simulink model "DIMR_ordinary"  (R2024b)
settings: Solver=daessc  StartTime=0.0  StopTime=60  RelTol=1e-3
values from neighbouring files (symbols this model uses):
  d_m0 = d_mn    (= 0)    [DIMR_main.m]
  d_m_cmd = 0.12787808985686    (= 0.127878089857)    [DIMR_main.m]
  dis_cmd = 0    [DIMR_main.m]
  jrk_cmd = 0.15    [DIMR_main.m]
  phi_cmd = 0*pi/180    (= 0)    [DIMR_main.m]
  ta = (vel_cmd-jrk_cmd*tt^2)/acc_cmd    (= 3.66666666667)    [DIMR_main.m]
  taz = z_vel_cmd/z_acc_cmd    (= 1.6)    [DIMR_main.m]
  tc = (x_cmd-2*(1/2*acc_cmd*ta^2+1/2*jrk_cmd*tt^2*ta+tt*vel_cmd))/vel_cmd    (= 10.6666666667)    [DIMR_main.m]
  tcz = (z_cmd-z_acc_cmd*taz^2)/z_vel_cmd    [DIMR_main.m]
  tcz2 = (z_cmd2-z_acc_cmd*taz^2)/z_vel_cmd    (= 0.9)    [DIMR_main.m]
  theta_f0 = -theta_p0    (= -0.024)    [DIMR_main.m]
  theta_f_cmd = 0.037940459    [DIMR_main.m]
  theta_p0 = theta_pn    (= 0.024)    [DIMR_main.m]
  theta_p_cmd = -0.037940459    [DIMR_main.m]
  ts = 15    [DIMR_main.m]
  ts2 = te+5    (= 39.3333333333)    [DIMR_main.m]
  tsz = 10    [DIMR_main.m]
  tsz2 = ts2    (= 39.3333333333)    [DIMR_main.m]
  tt = acc_cmd/jrk_cmd    (= 0.333333333333)    [DIMR_main.m]
  x_cmd = 3    [DIMR_main.m]
  z_0 = R_wo+L_bmy+L_my/2    [DIMR_main.m]
  z_acc_cmd = 0.05    [DIMR_main.m]
  z_cmd = 0.9-z_0    [DIMR_main.m]
  z_cmd2 = 0.9-0.7    (= 0.2)    [DIMR_main.m]
undefined symbols (not defined in the file or in its folder): Ac, Dc, DiscIntNeverNeededParam, dspblkCoreblockFVToolHelper, g, g_ext, g_fork, g_lift, g_reac, g_spado, g_yaw, gcbh, K_fd, K_fp, K_md, K_mp, K_pd, K_pp, K_wd, K_wi, K_wp, K_yd, K_yp, Kc, L_bg, L_bmx, L_bmy, L_bmz, L_bsx, L_bsy, L_bsz, L_by, L_ex, L_ey, L_ez, L_fg, L_fh, L_fx, L_fy, L_fz, L_lx, L_ly, L_lz, L_mg, L_mx, L_my, L_mz, L_wt, M_b, M_f, M_m, M_n11, M_n21, M_n22, M_n33, M_n44, Mc, N_f, N_w, omega_c ... (+10)
libraries: simulink x56, sm_lib x54, nesl_utility x12, slctrl_autotuning x1, slpidlib x1
(part 5 of 6)

== matlab function DIMR_ordinary/IK ==
  data: dz input; mass_l input; tau input; z input; ik_theta1 output; ik_delta2 output; ik_dtheta1 output; ik_ddelta2 output; ik_lt output
function [ik_theta1,ik_delta2,ik_dtheta1,ik_ddelta2,ik_lt] = IK(dz,mass_l,tau,z)
%#codegen

%    This function was generated by the Symbolic Math Toolbox version 24.2.
%    16-Apr-2025 15:03:47

% dz = complex(dz);  % if required to enforce complex operations
% mass_l = complex(mass_l);  % if required to enforce complex operations
% tau = complex(tau);  % if required to enforce complex operations
% z = complex(z);  % if required to enforce complex operations
t0 = roots([1.0,(mass_l.*3.312391896431465e+18-z.*1.104130632143822e+21-mass_l.*z.*4.416522528575287e+19+3.992701985426881e+20)./(tau.*2.251799813685248e+18+1.700361173501486e+19),0.0,-(mass_l.*-3.312391896431465e+18+z.*1.104130632143822e+21+mass_l.*z.*4.416522528575287e+19+2.336506037211149e+20)./(tau.*2.251799813685248e+18+1.700361173501486e+19),-1.0]);
t2 = real(t0(4));
t3 = atan(t2);
t4 = mass_l.^2;
t5 = mass_l.^3;
t7 = mass_l.^5;
t9 = t2.^2;
t10 = t2.^3;
t11 = tau.^2;
t12 = tau.^3;
t14 = tau.^5;
t16 = z.^2;
t17 = z.^3;
t19 = z.^5;
t22 = mass_l+2.5e+1;
t23 = -z;
t28 = mass_l.*z.*8.0e+3;
t30 = z.*2.0e+5;
t31 = mass_l+6.81e+2./1.0e+1;
t34 = tau.*5.62949953421312e+16;
t74 = mass_l.*tau.*3.614848010623563e+119;
t84 = mass_l.*1.568588020367706e+121;
t93 = tau.*1.348008262122411e+121;
t111 = tau.*z.*1.204949336874521e+122;
t116 = mass_l.*tau.*z.*9.823967899402039e+120;
t117 = z.*5.22862673455902e+123;
t120 = mass_l.*z.*3.628335485502499e+122;
t6 = t4.^2;
t8 = t4.^3;
t13 = t11.^2;
t15 = t11.^3;
t18 = t16.^2;
t20 = t16.^3;
t21 = t3.*2.0;
ik_theta1 = t21;
if nargout > 1
    t27 = 1.0./t22;
    t29 = -t28;
    t32 = -t30;
    t33 = 1.0./t31.^2;
    t36 = t34+4.250902933753714e+17;
    t42 = t14.*3.780256756564833e+113;
    t43 = t7.*1.98126031228264e+113;
    t51 = t4.*t12.*4.089923378308593e+113;
    t53 = t7.*z.*1.585008249826112e+115;
    t55 = mass_l.*t12.*2.044961689154296e+115;
    t56 = t5.*tau.*1.10623922643522e+115;
    t58 = t5.*t11.*7.325000484598409e+113;
    t62 = t12.*3.405637914264117e+117;
    t66 = t5.*3.162290386844749e+117;
    t70 = mass_l.*t12.*z.*5.453231171078124e+116;
    t71 = t5.*tau.*z.*5.899942540987838e+116;
    t80 = t4.*t11.*5.001176209735995e+116;
    t85 = t4.*t12.*z.*1.090646234215625e+115;
    t86 = t5.*t11.*z.*3.906666925119152e+115;
    t87 = t4.*2.305327187518337e+119;
    t88 = mass_l.*t11.*2.409025598810517e+118;
    t89 = t4.*tau.*7.506255827855932e+117;
    t90 = t12.*z.*6.816538963847654e+117;
    t92 = t7.*t16.*5.283360832753707e+116;
    t96 = t5.*z.*1.57648485563483e+119;
    t97 = t11.*8.666548343299187e+119;
    t107 = t12.*t16.*4.54435930923177e+118;
    t108 = t4.*tau.*z.*2.112292143405104e+119;
    t109 = t7.*t17.*9.392641480451035e+117;
    t112 = mass_l.*t12.*t16.*3.635487447385416e+117;
    t115 = t4.*z.*2.985248779870815e+120;
    t118 = t4.*t12.*t16.*7.270974894770831e+115;
    t122 = t7.*t19.*5.009408789573886e+119;
    t123 = mass_l.*t11.*z.*6.546151604904687e+119;
    t127 = -t111;
    t128 = t4.*t11.*z.*1.406896994108916e+118;
    t129 = t5.*t16.*tau.*1.179988508197568e+118;
    t133 = t11.*z.*8.030085329368392e+120;
    t134 = -t116;
    t135 = -t117;
    t138 = -t120;
    t142 = mass_l.*t16.*tau.*7.040973811350346e+121;
    t144 = mass_l.*t17.*tau.*6.555491712208709e+121;
    t146 = t5.*t17.*tau.*1.048878673953393e+119;
    t148 = t5.*t16.*2.712689641873518e+120;
    t150 = t17.*tau.*4.097182320130443e+122;
    t152 = t5.*t11.*t16.*7.813333850238303e+116;
    t155 = t11.*t16.*5.556862455262217e+121;
    t156 = t11.*t17.*2.712963142443855e+121;
    t157 = t4.*t16.*5.892258424926941e+121;
    t160 = mass_l.*t11.*t16.*4.68965664702972e+120;
    t161 = t4.*t16.*tau.*1.703191889319461e+120;
    t162 = mass_l.*t11.*t17.*4.340741027910169e+120;
    t163 = t4.*t17.*tau.*3.933295027325225e+120;
    t165 = mass_l.*t16.*9.950829266236052e+122;
    t166 = t16.*2.561474652798152e+124;
    t168 = t16.*tau.*8.340284253173257e+122;
    t171 = t5.*t11.*t17.*6.94518564465627e+117;
    t173 = t5.*t17.*1.4328795274517e+121;
    t179 = t17.*1.171218661794351e+125;
    t180 = mass_l.*t17.*1.751649839594256e+124;
    t188 = t4.*t11.*t16.*1.133264675661902e+119;
    t189 = t4.*t11.*t17.*2.604444616746101e+119;
    t191 = t5.*t19.*1.043626831161226e+123;
    t193 = t19.*8.153334618447079e+125;
    t198 = mass_l.*t19.*1.956800308427299e+125;
    t200 = t4.*t17.*9.042298806245061e+122;
    t203 = t4.*t19.*1.956800308427299e+124;
    t24 = cos(t21);
    t25 = sin(t21);
    t35 = t22.*6.0e+2+t29+t32+5.7323e+4;
    t38 = (t2.*t27.*t36)./1.104130632143822e+18;
    t39 = (t10.*t27.*t36)./1.104130632143822e+18;
    t40 = t8.*1.320840208188427e+111;
    t41 = t15.*8.343699359066055e+111;
    t44 = t6.*t11.*7.325000484598409e+111;
    t45 = t6.*tau.*1.10623922643522e+113;
    t46 = t8.*z.*1.056672166550741e+113;
    t47 = t4.*t13.*1.354078304772316e+112;
    t48 = mass_l.*t13.*6.770391523861579e+113;
    t50 = t6.*2.336765256726982e+115;
    t52 = t6.*tau.*z.*5.899942540987838e+114;
    t54 = t13.*1.079952046110396e+116;
    t59 = mass_l.*t13.*z.*1.805437739696421e+115;
    t61 = -t53;
    t64 = t4.*t13.*z.*3.610875479392842e+113;
    t65 = t6.*t11.*z.*3.906666925119152e+113;
    t67 = t8.*t16.*3.522240555169138e+114;
    t68 = t13.*z.*2.256797174620526e+116;
    t69 = t6.*z.*9.160647515406169e+116;
    t73 = -t62;
    t75 = t8.*t17.*6.261760986967357e+115;
    t78 = -t66;
    t81 = -t70;
    t82 = -t71;
    t91 = t8.*t18.*6.261760986967357e+116;
    t94 = t8.*t19.*3.339605859715924e+117;
    t95 = t13.*t16.*1.504531449747018e+117;
    t98 = -t85;
    t99 = -t86;
    t100 = mass_l.*t13.*t16.*1.203625159797614e+116;
    t101 = t6.*t16.*tau.*1.179988508197568e+116;
    t102 = -t90;
    t103 = t4.*t13.*t16.*2.407250319595228e+114;
    t104 = t6.*t11.*t16.*7.813333850238303e+114;
    t106 = t8.*t20.*7.421346354924275e+117;
    t110 = t6.*t16.*5.11289294892807e+117;
    t113 = t6.*t17.*tau.*1.048878673953393e+117;
    t114 = t6.*t18.*tau.*3.496262246511311e+117;
    t119 = t6.*t11.*t17.*6.94518564465627e+115;
    t121 = t6.*t17.*2.480721089402898e+119;
    t124 = -t108;
    t125 = -t109;
    t131 = t7.*t18.*9.392641480451035e+118;
    t132 = -t115;
    t137 = t6.*t11.*t18.*2.31506188155209e+116;
    t140 = -t122;
    t141 = t7.*t20.*1.113201953238641e+120;
    t143 = -t123;
    t145 = -t128;
    t147 = t5.*t18.*tau.*3.496262246511311e+119;
    t149 = -t133;
    t151 = t6.*t18.*4.740507646655564e+120;
    t153 = t6.*t19.*3.130880493483678e+121;
    t154 = t6.*t20.*6.957512207741508e+121;
    t158 = -t144;
    t159 = mass_l.*t18.*tau.*2.18516390406957e+122;
    t164 = -t146;
    t167 = -t148;
    t169 = -t150;
    t170 = t18.*tau.*1.365727440043481e+123;
    t172 = t5.*t11.*t18.*2.31506188155209e+118;
    t175 = -t156;
    t176 = t11.*t18.*9.043210474812851e+121;
    t177 = -t157;
    t178 = t5.*t18.*8.26907029800966e+121;
    t181 = mass_l.*t18.*3.392832413113396e+124;
    t182 = t4.*t18.*5.680992165475633e+122;
    t183 = -t162;
    t184 = -t163;
    t185 = mass_l.*t11.*t18.*1.446913675970056e+121;
    t186 = t4.*t18.*tau.*1.311098342441742e+121;
    t187 = t18.*2.884895378675286e+125;
    t190 = -t171;
    t192 = t5.*t20.*2.319170735913836e+123;
    t194 = t20.*1.811852137432684e+126;
    t199 = mass_l.*t20.*4.348445129838442e+125;
    t201 = -t189;
    t202 = t4.*t11.*t18.*8.681482055820337e+119;
    t204 = t4.*t20.*4.348445129838442e+124;
    t205 = -t191;
    t206 = -t193;
    t207 = -t198;
    t208 = -t203;
    t37 = (t9.*t27.*t35)./8.0e+3;
    ik_delta2 = -t37-t38-t39+z-1.89e+2./4.0e+2;
end
if nargout > 2
    t49 = -t46;
    t57 = -t50;
    t60 = -t52;
    t63 = -t54;
    t72 = -t59;
    t76 = -t64;
    t77 = -t65;
    t79 = -t68;
    t83 = -t75;
    t105 = -t94;
    t126 = -t110;
    t130 = -t113;
    t136 = -t119;
    t139 = -t121;
    t174 = -t153;
    t195 = -t181;
    t196 = -t182;
    t197 = -t187;
    t209 = t23+t37+t38+t39+1.89e+2./4.0e+2;
    et1 = t40+t41+t42+t43+t44+t45+t47+t48+t49+t51+t55+t56+t57+t58+t60+t61+t63+t67+t69+t72+t73+t74+t76+t77+t78+t79+t80+t81+t82+t83+t84+t87+t88+t89+t91+t92+t93+t95+t96+t97+t98+t99+t100+t101+t102+t103+t104+t105+t106+t107+t112+t114+t118+t124+t125+t126+t127+t129+t130+t131+t132+t134+t135+t136+t137+t138+t139+t140+t141+t142+t143+t145+t147+t149+t151+t152+t154+t155+t158+t159+t160+t161+t164+t165+t166+t167+t168+t169+t170+t172+t173+t174+t175+t176+t177+t178+t179+t180+t183+t184+t185+t186+t188+t190+t192+t194+t195+t196+t197+t199+t200+t201+t202+t204+t205+t206+t207+t208;
    et2 = -7.606317967206997e+122;
    t210 = et1+et2;
    t211 = 1.0./t210;
    et3 = mass_l.*-8.341180644416429e+99;
    et4 = t2.*-3.484897789398941e+102;
    et5 = t4.*1.116786520175198e+98+t5.*1.787461437567226e+96;
    et6 = t6.*6.140861299659515e+93;
    et7 = t9.*2.005754656158809e+102;
    et8 = t10.*9.179678600785833e+100;
    et9 = t11.*6.768174067705626e+96+t12.*2.987712913028659e+95;
    et10 = t16.*1.240873911305775e+103;
    et11 = t17.*-6.620227546545282e+103;
    et12 = t18.*7.581310246493228e+103;
    et13 = tau.*-1.004147809508344e+101;
    et14 = z.*2.78039354813881e+102;
    et15 = mass_l.*t2.*1.127177973099862e+100;
    et16 = mass_l.*t9.*6.373446754820384e+100;
    et17 = mass_l.*t10.*1.878106750040951e+99;
    et18 = mass_l.*t11.*-1.131163232401083e+97;
    et19 = mass_l.*t12.*-4.993357089194394e+95;
    et20 = mass_l.*t16.*1.588519608233696e+102;
    et21 = mass_l.*t17.*-8.854030285433525e+102;
    et22 = mass_l.*t18.*1.213009639438916e+103;
    et23 = mass_l.*tau.*-1.161571865623982e+99;
    et24 = mass_l.*z.*3.676330724720587e+100;
    et25 = t2.*t4.*1.050729864818058e+99;
    et26 = t2.*t5.*9.564633586316173e+95-t2.*t6.*8.794125430247251e+94;
    et27 = t2.*t7.*-3.987572272506178e+92-t2.*t11.*1.530222009440098e+98;
    et28 = t4.*t9.*7.896768589768845e+98;
    et29 = t2.*t12.*2.480546600446387e+96;
    et30 = t4.*t10.*1.677511635877758e+97;
    et31 = t5.*t9.*4.543602806080409e+96+t2.*t13.*8.212511641306701e+94;
    et32 = t4.*t11.*3.405545327663178e+94+t5.*t10.*6.304617600983768e+94;
    et33 = t6.*t9.*1.023476883276586e+94+t4.*t12.*1.503328911103625e+93;
    et34 = t2.*t16.*1.16747762757562e+104;
    et35 = t2.*t17.*-3.542456883820805e+103;
    et36 = t2.*t18.*-1.085694497561389e+105;
    et37 = t4.*t16.*7.161352844912477e+100;
    et38 = t9.*t11.*-6.676607447632182e+98;
    et39 = t2.*t19.*1.640976243829703e+105;
    et40 = t4.*t17.*-4.26941789783676e+101;
    et41 = t5.*t16.*1.280825369351028e+99;
    et42 = t9.*t12.*-2.876866570872632e+97;
    et43 = t10.*t11.*1.568816837840201e+99;
    et44 = t4.*t18.*7.278057836633499e+101;
    et45 = t5.*t17.*-8.60378033176908e+99;
    et46 = t6.*t16.*6.550252052970149e+96+t9.*t13.*6.994880150221821e+94;
    et47 = t10.*t12.*-4.354804437206384e+96;
    et48 = t5.*t18.*1.940815423102266e+100;
    et49 = t6.*t17.*-5.822446269306799e+97+t9.*t14.*1.852673427797059e+93;
    et50 = t10.*t13.*-1.441774249664796e+95;
    et51 = t6.*t18.*1.940815423102266e+98;
    et52 = t9.*t16.*8.774187321965383e+103;
    et53 = t9.*t17.*-1.682815854103855e+104;
    et54 = t10.*t16.*1.863901817641953e+102;
    et55 = t9.*t18.*1.263551707748871e+104;
    et56 = t10.*t17.*-2.335043555919914e+102;
    et57 = t11.*t16.*3.783939252959087e+99;
    et58 = t12.*t16.*1.670365456781806e+98;
    et59 = tau.*t2.*-2.593856817883973e+99;
    et60 = t4.*tau.*1.496111738184045e+97+t5.*tau.*2.367147283065111e+95;
    et61 = t6.*tau.*8.132384193391584e+92;
    et62 = t9.*tau.*2.622463267042749e+101;
    et63 = t10.*tau.*2.418926682338227e+100;
    et64 = t16.*tau.*1.66234637576005e+102;
    et65 = t17.*tau.*-8.767212159500411e+102;
    et66 = t18.*tau.*1.003998048566862e+103;
    et67 = z.*t2.*-3.757259910332874e+102;
    et68 = t4.*z.*-4.765558824701087e+99;
    et69 = t5.*z.*-7.968627256890173e+97;
    et70 = t6.*z.*-3.275126026485075e+95;
    et71 = t9.*z.*-2.124482251606795e+103;
    et72 = t10.*z.*-6.260355833469838e+101;
    et73 = t11.*z.*3.770544108003612e+99;
    et74 = t12.*z.*1.664452363064798e+98;
    et75 = tau.*z.*3.871906218746606e+101;
    et76 = mass_l.*t2.*t11.*-1.328598509782306e+97;
    et77 = mass_l.*t2.*t12.*2.057890242755185e+94+mass_l.*t2.*t13.*6.813194951514761e+92;
    et78 = mass_l.*t2.*t16.*9.658642140148833e+102;
    et79 = mass_l.*t2.*t17.*8.777385710151702e+102;
    et80 = mass_l.*t2.*t18.*-1.983257632672678e+104;
    et81 = mass_l.*t9.*t11.*3.973136215607041e+96;
    et82 = mass_l.*t2.*t19.*3.281952487659406e+104;
    et83 = mass_l.*t9.*t12.*1.753883729620896e+95;
    et84 = mass_l.*t10.*t11.*3.352074536750164e+97;
    et85 = mass_l.*t10.*t12.*6.173670728265554e+94+mass_l.*t10.*t13.*2.043958485454428e+93;
    et86 = mass_l.*t9.*t16.*8.533884126265777e+102;
    et87 = mass_l.*t9.*t17.*-2.171005229854491e+103;
    et88 = mass_l.*t10.*t16.*1.701275374146355e+101;
    et89 = mass_l.*t9.*t18.*2.021682732398194e+103;
    et90 = mass_l.*t10.*t17.*-2.802052267103897e+101;
    et91 = mass_l.*t11.*t16.*3.027151402367269e+98;
    et92 = mass_l.*t12.*t16.*1.336292365425445e+97;
    et93 = mass_l.*tau.*t2.*-2.02994943064197e+98;
    et94 = mass_l.*t9.*tau.*8.460399773172835e+99;
    et95 = mass_l.*t10.*tau.*4.991979924562494e+98;
    et96 = mass_l.*t16.*tau.*2.118926194963077e+101;
    et97 = mass_l.*t17.*tau.*-1.172545224968073e+102;
    et98 = mass_l.*t18.*tau.*1.606396877706979e+102;
    et99 = mass_l.*z.*t2.*-8.50776972958687e+101;
    et100 = mass_l.*t9.*z.*-1.376244139960641e+102;
    et101 = mass_l.*t10.*z.*-3.622483423973107e+100;
    et102 = mass_l.*t11.*z.*1.281181288023899e+98;
    et103 = mass_l.*t12.*z.*5.655590178190109e+96;
    et104 = mass_l.*tau.*z.*5.513546620426123e+99;
    et105 = t2.*t4.*t11.*2.540546642850375e+95-t2.*t5.*t11.*3.685655116518591e+92;
    et106 = t2.*t4.*t16.*1.53674607107294e+101;
    et107 = t2.*t4.*t17.*1.541050008009675e+102;
    et108 = t2.*t5.*t16.*-4.623150024029024e+99;
    et109 = t2.*t4.*t18.*-1.436101016178062e+103;
    et110 = t2.*t5.*t17.*7.799137408725148e+100;
    et111 = t2.*t6.*t16.*-1.292490914560256e+98;
    et112 = t4.*t9.*t11.*7.946272431214082e+94;
    et113 = t2.*t4.*t19.*2.625561990127525e+103;
    et114 = t2.*t5.*t18.*-5.142383704871928e+101;
    et115 = t2.*t6.*t17.*1.542715111461578e+99;
    et116 = t2.*t7.*t16.*-7.089017373344317e+95+t4.*t9.*t12.*3.507767459241792e+93;
    et117 = t4.*t10.*t11.*2.942000483658635e+95;
    et118 = t2.*t5.*t19.*1.05022479605101e+102;
    et119 = t2.*t6.*t18.*-9.080726690063216e+99;
    et120 = t2.*t7.*t17.*9.45202316445909e+96+t5.*t10.*t11.*1.105696534955577e+93;
    et121 = t2.*t6.*t19.*2.10044959210202e+100;
    et122 = t2.*t7.*t18.*-6.30134877630606e+97;
    et123 = t2.*t7.*t19.*1.680359673681616e+98;
    et124 = t2.*t11.*t16.*2.822829603167083e+100;
    et125 = t4.*t9.*t16.*2.683729178687676e+101;
    et126 = t2.*t11.*t17.*1.365057450562441e+100;
    et127 = t4.*t9.*t17.*-9.89703055885688e+101;
    et128 = t4.*t10.*t16.*4.663474268489463e+99;
    et129 = t5.*t9.*t16.*2.969109167657064e+99;
    et130 = t4.*t9.*t18.*1.213009639438916e+102;
    et131 = t4.*t10.*t17.*-1.120820906841559e+100;
    et132 = t4.*t11.*t16.*6.054302804734539e+96;
    et133 = t5.*t9.*t17.*-1.804807930289817e+100;
    et134 = t5.*t10.*t16.*3.362462720524677e+97;
    et135 = t6.*t9.*t16.*1.091708675495025e+97;
    et136 = t4.*t12.*t16.*2.672584730850889e+95;
    et137 = t5.*t9.*t18.*3.234692371837111e+100;
    et138 = t5.*t10.*t17.*-1.494427875788745e+98;
    et139 = t6.*t9.*t17.*-9.704077115511332e+97;
    et140 = t6.*t9.*t18.*3.234692371837111e+98;
    et141 = t9.*t11.*t16.*8.829191590237869e+99;
    et142 = t9.*t12.*t16.*3.897519399157546e+98;
    et143 = t10.*t11.*t16.*3.268889426287372e+100;
    et144 = t10.*t11.*t17.*-4.095172351687323e+100;
    et145 = t2.*t4.*tau.*3.836794767206729e+96-t2.*t5.*tau.*5.566165181254684e+93;
    et146 = t4.*t9.*tau.*1.049774627912272e+98;
    et147 = t4.*t10.*tau.*4.443080032632926e+96;
    et148 = t5.*t9.*tau.*6.017123956743121e+95+t5.*t10.*tau.*1.669849554376405e+94;
    et149 = t6.*t9.*tau.*1.355397365565264e+93;
    et150 = t2.*t16.*tau.*4.263105296896365e+101;
    et151 = t2.*t17.*tau.*2.061542659723957e+101;
    et152 = t4.*t16.*tau.*9.514305902282482e+99;
    et153 = t4.*t17.*tau.*-5.654019026496479e+100;
    et154 = t5.*t16.*tau.*1.696205707948944e+98;
    et155 = t4.*t18.*tau.*9.638381266241877e+100;
    et156 = t5.*t17.*tau.*-1.139404454182539e+99;
    et157 = t6.*t16.*tau.*8.674543139617689e+95;
    et158 = t5.*t18.*tau.*2.570235004331167e+99;
    et159 = t6.*t17.*tau.*-7.710705012993501e+96;
    et160 = t6.*t18.*tau.*2.570235004331167e+97;
    et161 = t9.*t16.*tau.*1.166416253235857e+103;
    et162 = t9.*t17.*tau.*-2.228564428423378e+103;
    et163 = t10.*t16.*tau.*4.936755591814363e+101;
    et164 = t9.*t18.*tau.*1.67333008094477e+103;
    et165 = t10.*t17.*tau.*-6.184627979171871e+101;
    et166 = t2.*t4.*z.*-2.89759264204465e+100;
    et167 = t2.*t5.*z.*7.899647139136532e+97;
    et168 = t2.*t6.*z.*5.35479560821623e+96+t2.*t7.*z.*2.658381515004119e+94;
    et169 = t2.*t11.*z.*4.428661699274352e+99;
    et170 = t4.*t9.*z.*-2.560165237879733e+100;
    et171 = t2.*t12.*z.*-6.859634142517282e+96;
    et172 = t4.*t10.*z.*-5.103826122439064e+98;
    et173 = t5.*t9.*z.*-1.953904706869042e+98;
    et174 = t2.*t13.*z.*-2.271064983838254e+95;
    et175 = t4.*t11.*z.*-9.081454207101808e+95;
    et176 = t5.*t10.*z.*-2.521847040393507e+96;
    et177 = t6.*t9.*z.*-5.458543377475124e+95;
    et178 = t4.*t12.*z.*-4.008877096276334e+94;
    et179 = t9.*t11.*z.*-1.32437873853568e+99;
    et180 = t9.*t12.*z.*-5.84627909873632e+97;
    et181 = t10.*t11.*z.*-1.117358178916721e+100;
    et182 = t10.*t12.*z.*-2.057890242755185e+97;
    et183 = t10.*t13.*z.*-6.813194951514761e+95;
    et184 = tau.*z.*t2.*6.7664981021399e+100;
    et185 = t4.*tau.*z.*-6.356778584889232e+98;
    et186 = t5.*tau.*z.*-1.055290702471265e+97;
    et187 = t6.*tau.*z.*-4.337271569808845e+94;
    et188 = t9.*tau.*z.*-2.820133257724278e+102;
    et189 = t10.*tau.*z.*-1.663993308187498e+101;
    et190 = mass_l.*t2.*t11.*t16.*2.135408511983047e+99;
    et191 = mass_l.*t2.*t11.*t17.*1.638068940674929e+99;
    et192 = mass_l.*t9.*t11.*t16.*7.063353272190295e+98;
    et193 = mass_l.*t9.*t12.*t16.*3.118015519326037e+97;
    et194 = mass_l.*t10.*t11.*t16.*2.983677052681757e+99;
    et195 = mass_l.*t10.*t11.*t17.*-4.914206822024788e+99;
    et196 = mass_l.*t2.*t16.*tau.*3.224945398141936e+100;
    et197 = mass_l.*t2.*t17.*tau.*2.473851191668748e+100;
    et198 = mass_l.*t9.*t16.*tau.*1.13370380114679e+102;
    et199 = mass_l.*t9.*t17.*tau.*-2.875076923821426e+102;
    et200 = mass_l.*t10.*t16.*tau.*4.506020991576958e+100;
    et201 = mass_l.*t9.*t18.*tau.*2.677328129511632e+102;
    et202 = mass_l.*t10.*t17.*tau.*-7.421553575006245e+100;
    et203 = mass_l.*t2.*t11.*z.*7.776691780949094e+96;
    et204 = mass_l.*t2.*t12.*z.*-2.743853657006913e+95;
    et205 = mass_l.*t2.*t13.*z.*-9.084259935353014e+93;
    et206 = mass_l.*t9.*t11.*z.*-1.059502990828544e+98;
    et207 = mass_l.*t9.*t12.*z.*-4.677023278989056e+96;
    et208 = mass_l.*t10.*t11.*z.*-6.430766371439309e+98;
    et209 = mass_l.*t10.*t12.*z.*-8.231560971020738e+95;
    et210 = mass_l.*t10.*t13.*z.*-2.725277980605904e+94;
    et211 = mass_l.*tau.*z.*t2.*1.48736062718141e+98;
    et212 = mass_l.*t9.*tau.*z.*-1.827903055031226e+101;
    et213 = mass_l.*t10.*tau.*z.*-9.618026587838609e+99;
    et214 = t2.*t4.*t11.*t16.*3.533686000662376e+97;
    et215 = t2.*t4.*t11.*t17.*6.552275762699717e+97;
    et216 = t2.*t5.*t11.*t16.*-1.965682728809915e+95;
    et217 = t2.*t5.*t11.*t17.*8.736367683599623e+95;
    et218 = t4.*t9.*t11.*t16.*1.412670654438059e+97;
    et219 = t4.*t9.*t12.*t16.*6.236031038652074e+95;
    et220 = t4.*t10.*t11.*t16.*8.178747175274668e+97;
    et221 = t4.*t10.*t11.*t17.*-1.965682728809915e+98;
    et222 = t5.*t10.*t11.*t16.*5.897048186429746e+95;
    et223 = t5.*t10.*t11.*t17.*-2.620910305079887e+96;
    et224 = t2.*t4.*t16.*tau.*5.336657760032935e+98;
    et225 = t2.*t4.*t17.*tau.*9.895404766674994e+98;
    et226 = t2.*t5.*t16.*tau.*-2.968621430002498e+96;
    et227 = t2.*t5.*t17.*tau.*1.319387302223332e+97;
    et228 = t4.*t9.*t16.*tau.*3.561192218013222e+100;
    et229 = t4.*t9.*t17.*tau.*-1.310670457299268e+101;
    et230 = t4.*t10.*t16.*tau.*1.235174109190673e+99;
    et231 = t5.*t9.*t16.*tau.*3.932011371897805e+98;
    et232 = t4.*t9.*t18.*tau.*1.606396877706979e+101;
    et233 = t4.*t10.*t17.*tau.*-2.968621430002498e+99;
    et234 = t5.*t9.*t17.*tau.*-2.39011936081515e+99;
    et235 = t5.*t10.*t16.*tau.*8.905864290007494e+96;
    et236 = t6.*t9.*t16.*tau.*1.445757189936282e+96;
    et237 = t5.*t9.*t18.*tau.*4.283725007218612e+99;
    et238 = t5.*t10.*t17.*tau.*-3.958161906669997e+97;
    et239 = t6.*t9.*t17.*tau.*-1.285117502165584e+97;
    et240 = t6.*t9.*t18.*tau.*4.283725007218612e+97;
    et241 = t2.*t4.*t11.*z.*-6.406225535949141e+96;
    et242 = t2.*t5.*t11.*z.*1.474262046607436e+94;
    et243 = t4.*t9.*t11.*z.*-2.119005981657089e+96;
    et244 = t4.*t9.*t12.*z.*-9.354046557978112e+94;
    et245 = t4.*t10.*t11.*z.*-8.95103115804527e+96;
    et246 = t5.*t10.*t11.*z.*-4.422786139822309e+94;
    et247 = t2.*t4.*tau.*z.*-9.674836194425808e+97;
    et248 = t2.*t5.*tau.*z.*2.226466072501874e+95;
    et249 = t4.*t9.*tau.*z.*-3.401111403440369e+99;
    et250 = t4.*t10.*tau.*z.*-1.351806297473088e+98;
    et251 = t5.*t9.*tau.*z.*-2.587569231439284e+97;
    et252 = t5.*t10.*tau.*z.*-6.679398217505621e+95;
    et253 = t6.*t9.*tau.*z.*-7.228785949681408e+94;
    et254 = -7.585013891843565e+101;
    et255 = et3+et4+et5+et6+et7+et8+et9+et10+et11+et12+et13+et14+et15+et16+et17+et18+et19+et20+et21+et22+et23+et24+et25+et26+et27+et28+et29+et30+et31+et32+et33+et34+et35+et36+et37+et38+et39+et40+et41+et42+et43+et44+et45+et46+et47+et48+et49+et50+et51+et52+et53+et54+et55+et56+et57+et58+et59+et60+et61+et62+et63+et64+et65+et66+et67+et68+et69+et70+et71+et72+et73+et74+et75+et76+et77+et78+et79+et80+et81+et82+et83+et84+et85+et86+et87+et88+et89+et90+et91+et92+et93+et94+et95+et96+et97+et98+et99+et100+et101+et102+et103+et104+et105+et106+et107+et108+et109+et110+et111+et112+et113+et114+et115+et116+et117+et118+et119+et120+et121+et122+et123+et124+et125+et126+et127+et128+et129+et130+et131+et132+et133+et134+et135+et136+et137+et138+et139+et140+et141+et142+et143+et144+et145+et146+et147+et148+et149+et150+et151+et152+et153+et154+et155+et156+et157+et158+et159+et160+et161+et162+et163+et164+et165+et166+et167+et168+et169+et170+et171+et172+et173+et174+et175+et176+et177+et178+et179+et180+et181+et182+et183+et184+et185+et186+et187+et188+et189+et190+et191+et192+et193+et194+et195+et196+et197+et198+et199+et200+et201+et202;
    et256 = et203+et204+et205+et206+et207+et208+et209+et210+et211+et212+et213+et214+et215+et216+et217+et218+et219+et220+et221+et222+et223+et224+et225+et226+et227+et228+et229+et230+et231+et232+et233+et234+et235+et236+et237+et238+et239+et240+et241+et242+et243+et244+et245+et246+et247+et248+et249+et250+et251+et252+et253+et254;
    ik_dtheta1 = dz.*t22.*t211.*(et255+et256).*4.416522528575287e+19;
end
if nargout > 3
    et257 = mass_l.*2.639612829107319e+105;
    et258 = t2.*-2.425916942554274e+106;
    et259 = t4.*3.923391393236826e+103;
    et260 = t5.*-5.861747496028786e+101;
    et261 = t6.*-4.257988015416612e+99;
    et262 = t7.*3.588815045255561e+97+t8.*2.392543363503707e+95;
    et263 = t9.*2.489404006316541e+107;
    et264 = t10.*1.063508391175204e+106;
    et265 = t11.*6.062497748591897e+103;
    et266 = t12.*-2.099683475413849e+101;
    et267 = t13.*-6.95156260390047e+99;
    et268 = t16.*4.35932377026314e+108;
    et269 = t17.*2.171017591121773e+109;
    et270 = t18.*-5.256775327674829e+109;
    et271 = t19.*-1.476878619446733e+110;
    et272 = t20.*3.281952487659406e+110;
    et273 = tau.*9.395175677405263e+104;
    et274 = z.*-8.798709430357731e+107;
    et275 = mass_l.*t2.*-6.111698685858886e+104;
    et276 = mass_l.*t9.*1.27829334016942e+105;
    et277 = mass_l.*t10.*-3.264288195402587e+103;
    et278 = mass_l.*t11.*8.0303147124868e+101;
    et279 = mass_l.*t12.*1.234734145653111e+99;
    et280 = mass_l.*t13.*4.087916970908856e+97;
    et281 = mass_l.*t16.*1.533543184200916e+107;
    et282 = mass_l.*t17.*3.236034148667107e+108;
    et283 = mass_l.*t18.*-6.195522595109628e+108;
    [ik_ddelta2,ik_lt] = ft_1({dz,et257,et258,et259,et260,et261,et262,et263,et264,et265,et266,et267,et268,et269,et270,et271,et272,et273,et274,et275,et276,et277,et278,et279,et280,et281,et282,et283,mass_l,t10,t11,t12,t13,t14,t16,t17,t18,t19,t2,t20,t209,t211,t24,t25,t33,t4,t5,t6,t7,t8,t9,tau,z}, nargout);
end
end
function [ik_ddelta2,ik_lt] = ft_1(ct, nargout)
ik_ddelta2 = 0;
ik_lt = 0;
[dz,et257,et258,et259,et260,et261,et262,et263,et264,et265,et266,et267,et268,et269,et270,et271,et272,et273,et274,et275,et276,et277,et278,et279,et280,et281,et282,et283,mass_l,t10,t11,t12,t13,t14,t16,t17,t18,t19,t2,t20,t209,t211,t24,t25,t33,t4,t5,t6,t7,t8,t9,tau,z] = ct{:};
et284 = mass_l.*t19.*-3.544508686672159e+109;
et285 = mass_l.*t20.*7.876685970382575e+109;
et286 = mass_l.*tau.*1.198676715771426e+103;
et287 = mass_l.*z.*-6.135078034300976e+106;
et288 = t2.*t4.*1.4286014167529e+102;
et289 = t2.*t5.*1.114446801392038e+101;
et290 = t2.*t6.*7.402091862921251e+98;
et291 = t2.*t7.*1.228172259931903e+96;
et292 = t2.*t11.*2.118445374560911e+102;
et293 = t4.*t9.*-8.260916274751945e+103;
et294 = t2.*t12.*7.861260986891366e+100;
et295 = t4.*t10.*-3.258788008708109e+102;
et296 = t5.*t9.*-6.95829447816559e+101;
et297 = t2.*t13.*-1.480221562989191e+99;
et298 = t4.*t11.*4.585290937721163e+100;
et299 = t5.*t10.*-2.751724922475081e+99;
et300 = t6.*t9.*5.824125025344651e+99;
et301 = t2.*t14.*-3.920534874232747e+97;
et302 = t4.*t12.*2.469468291306221e+97;
et303 = t5.*t11.*-1.016898046233295e+98;
et304 = t6.*t10.*2.708590632516153e+98;
et305 = t7.*t9.*8.160407152792994e+97;
et306 = t4.*t13.*8.175833941817713e+95+t6.*t11.*8.845572279644618e+95;
et307 = t7.*t10.*1.228172259931903e+96+t8.*t9.*2.392543363503707e+95;
et308 = t2.*t16.*1.587334907503222e+107;
et309 = t2.*t17.*-4.127580745896436e+108;
et310 = t2.*t18.*9.138385015952162e+108;
et311 = t4.*t16.*-1.149506730060015e+106;
et312 = t9.*t11.*-3.985307324265062e+103;
et313 = t2.*t19.*-5.054206830995485e+108;
et314 = t4.*t17.*1.66614501517342e+107;
et315 = t5.*t16.*-4.998435045520261e+104;
et316 = t9.*t12.*1.818544799899849e+101;
et317 = t10.*t11.*-3.345064469954305e+102;
et318 = t4.*t18.*-1.058932042061658e+107;
et319 = t5.*t17.*2.645099503722557e+105;
et320 = t6.*t16.*-9.530388378554919e+101;
et321 = t9.*t13.*6.020777975599281e+99;
et322 = t10.*t12.*-1.221961057016e+101;
et323 = t4.*t19.*-3.544508686672159e+108;
et324 = t5.*t18.*1.489872465452971e+106;
et325 = t6.*t17.*-4.469617396358912e+103;
et326 = t7.*t16.*9.570173454014828e+100;
et327 = t10.*t13.*2.529453585522464e+99;
et328 = t4.*t20.*7.876685970382575e+108;
et329 = t5.*t19.*-1.890404632891818e+107;
et330 = t6.*t18.*8.578889838797288e+104;
et331 = t7.*t17.*-1.701364169602636e+102;
et332 = t8.*t16.*6.380115636009885e+98;
et333 = t10.*t14.*6.699545015928335e+97;
et334 = t5.*t20.*4.20089918420404e+107;
et335 = t6.*t19.*-5.671213898675454e+105;
et336 = t7.*t18.*1.701364169602636e+103;
et337 = t8.*t17.*-1.134242779735091e+100;
et338 = t9.*t16.*-9.178795860835495e+108;
et339 = t6.*t20.*1.260269755261212e+106;
et340 = t7.*t19.*-9.073942237880726e+103;
et341 = t8.*t18.*1.134242779735091e+101;
et342 = t9.*t17.*2.577146103024293e+109;
et343 = t10.*t16.*-3.620875565231232e+107;
et344 = t7.*t20.*2.016431608417939e+104;
et345 = t8.*t19.*-6.049294825253817e+101;
et346 = t9.*t18.*7.190277809067471e+109;
et347 = t10.*t17.*1.019157378694475e+107;
et348 = t11.*t16.*5.09476770857907e+105;
et349 = t8.*t20.*1.344287738945293e+102;
et350 = t9.*t19.*-3.358192243947734e+110;
et351 = t10.*t18.*3.343939052489078e+108;
et352 = t11.*t17.*3.766289060123314e+105;
et353 = t12.*t16.*2.743853657006913e+102;
et354 = t9.*t20.*3.281952487659406e+110;
et355 = t10.*t19.*-5.054206830995485e+108;
et356 = t11.*t18.*1.092045960449953e+106;
et357 = t13.*t16.*9.084259935353014e+100;
et358 = tau.*t2.*-3.201653899884155e+105;
et359 = t4.*tau.*6.896655349324523e+101;
et360 = t5.*tau.*-1.535743936664436e+99;
et361 = t6.*tau.*1.335879643501124e+97;
et362 = t9.*tau.*-6.226091909409972e+104;
et363 = t10.*tau.*1.390991195047167e+105;
et364 = t16.*tau.*7.662950388138359e+106;
et365 = t17.*tau.*5.687940506164578e+106;
et366 = t18.*tau.*1.649234127779166e+107;
et367 = z.*t2.*2.037232895286295e+107;
et368 = t4.*z.*-4.600629552602749e+104;
et369 = t5.*z.*2.912430733800396e+103;
et370 = t6.*z.*1.672791100679599e+101;
et371 = t7.*z.*-2.871052036204448e+99;
et372 = t8.*z.*-1.914034690802966e+97;
et373 = t9.*z.*-4.260977800564734e+107;
et374 = t10.*z.*1.088096065134196e+106;
et375 = t11.*z.*-2.676771570828933e+104;
et376 = t12.*z.*-4.115780485510369e+101;
et377 = t13.*z.*-1.362638990302952e+100;
et378 = tau.*z.*-3.995589052571419e+105;
et379 = mass_l.*t2.*t11.*-4.455890487678097e+101;
et380 = mass_l.*t2.*t12.*-1.945860973394936e+100;
et381 = mass_l.*t2.*t13.*2.098464045066546e+97;
et382 = mass_l.*t2.*t14.*5.558020283391177e+95;
et383 = mass_l.*t2.*t16.*4.98469059730937e+106;
et384 = mass_l.*t2.*t17.*-6.049703096989982e+107;
et385 = mass_l.*t2.*t18.*1.537954705017278e+108;
et386 = mass_l.*t9.*t11.*1.115137400075502e+102;
et387 = mass_l.*t2.*t19.*-1.010841366199097e+108;
et388 = mass_l.*t9.*t12.*-1.124554702055998e+99;
et389 = mass_l.*t10.*t11.*2.353636634110694e+101;
et390 = mass_l.*t9.*t13.*-3.723138513204756e+97;
et391 = mass_l.*t10.*t12.*1.060106649462622e+100;
et392 = mass_l.*t10.*t13.*2.098464045066546e+97;
et393 = mass_l.*t10.*t14.*5.558020283391177e+95;
et394 = mass_l.*t9.*t16.*-9.662468181390259e+107;
et395 = mass_l.*t9.*t17.*2.229741986541055e+108;
et396 = mass_l.*t10.*t16.*-2.988424616267488e+106;
et397 = mass_l.*t9.*t18.*1.654173286042955e+109;
et398 = mass_l.*t10.*t17.*-2.789738008553524e+106;
et399 = mass_l.*t11.*t16.*3.736848151452158e+104;
et400 = mass_l.*t9.*t19.*-7.307135935674161e+109;
et401 = mass_l.*t10.*t18.*6.108433508631848e+107;
et402 = mass_l.*t11.*t17.*3.209091719608034e+104;
et403 = mass_l.*t12.*t16.*2.19508292560553e+101;
et404 = mass_l.*t9.*t20.*7.876685970382575e+109;
et405 = mass_l.*t10.*t19.*-1.010841366199097e+108;
et406 = mass_l.*t11.*t18.*1.747273536719925e+105;
et407 = mass_l.*t13.*t16.*7.267407948282412e+99;
et408 = mass_l.*tau.*t2.*-8.318558928291235e+103;
et409 = mass_l.*t9.*tau.*1.696931667960436e+103;
et410 = mass_l.*t10.*tau.*-3.142898118320109e+102;
et411 = mass_l.*t16.*tau.*5.618445664955875e+105;
et412 = mass_l.*t17.*tau.*4.846447654062495e+105;
et413 = mass_l.*t18.*tau.*2.638774604446665e+106;
et414 = mass_l.*z.*t2.*7.196530636643248e+105;
et415 = mass_l.*t9.*z.*3.802886396275403e+106;
et416 = mass_l.*t10.*z.*2.607763765192417e+105;
et417 = mass_l.*t11.*z.*-4.127569253479015e+103;
et418 = mass_l.*t12.*z.*-3.292624388408295e+100;
et419 = mass_l.*t13.*z.*-1.090111192242362e+99;
et420 = mass_l.*tau.*z.*-6.196005853911583e+104;
et421 = t2.*t4.*t11.*-2.231937648661653e+99;
et422 = t2.*t4.*t12.*-9.852567128554641e+97;
et423 = t2.*t5.*t11.*1.362218131065271e+97;
et424 = t2.*t5.*t12.*6.0133156444145e+95;
et425 = t2.*t4.*t16.*3.719304513107366e+105;
et426 = t2.*t4.*t17.*-3.34265406180636e+106;
et427 = t2.*t5.*t16.*1.002796218541908e+104;
et428 = t2.*t4.*t18.*9.985859254752992e+106;
et429 = t2.*t5.*t17.*-8.451215784309677e+104;
et430 = t2.*t6.*t16.*8.987273329277693e+101;
et431 = t4.*t9.*t11.*-7.49502403837478e+99;
et432 = t2.*t4.*t19.*-8.086730929592777e+106;
et433 = t2.*t5.*t18.*3.067232347747103e+105;
et434 = t2.*t6.*t17.*-9.20169704324131e+102;
et435 = t2.*t7.*t16.*2.18341735099005e+99;
et436 = t4.*t9.*t12.*2.469468291306221e+97;
et437 = t4.*t10.*t11.*-3.533378147445895e+99;
et438 = t5.*t9.*t11.*-5.943524297449045e+97;
et439 = t2.*t5.*t19.*-3.234692371837111e+105;
et440 = t2.*t6.*t18.*4.28024198718602e+103;
et441 = t2.*t7.*t17.*-2.9112231346534e+100;
et442 = t4.*t9.*t13.*8.175833941817713e+95;
et443 = t4.*t10.*t12.*-1.559758867330085e+98;
et444 = t5.*t10.*t11.*1.362218131065271e+97;
et445 = t6.*t9.*t11.*8.845572279644618e+95;
et446 = t2.*t6.*t19.*-6.469384743674221e+103;
et447 = t2.*t7.*t18.*1.940815423102266e+101;
et448 = t5.*t10.*t12.*6.0133156444145e+95;
et449 = t2.*t7.*t19.*-5.175507794939377e+101;
et450 = t2.*t11.*t16.*-2.479930720735169e+104;
et451 = t4.*t9.*t16.*-2.935877530221527e+106;
et452 = t2.*t11.*t17.*-5.045252337278782e+104;
et453 = t2.*t12.*t16.*-1.094729680950516e+103;
et454 = t4.*t9.*t17.*-1.006071770093514e+106;
et455 = t4.*t10.*t16.*-4.721467128685891e+104;
et456 = t5.*t9.*t16.*3.018215310280541e+103;
et457 = t2.*t12.*t17.*-2.227153942375741e+103;
et458 = t4.*t9.*t18.*1.540539166801335e+108;
et459 = t4.*t10.*t17.*-4.780955308600518e+105;
et460 = t4.*t11.*t16.*6.0296050290807e+102;
et461 = t5.*t9.*t17.*-6.296299569884477e+105;
et462 = t5.*t10.*t16.*1.434286592580155e+103;
et463 = t6.*t9.*t16.*1.386485250121202e+103;
et464 = t4.*t9.*t19.*-6.554610485873761e+108;
et465 = t4.*t10.*t18.*4.423191129828431e+106;
et466 = t4.*t11.*t17.*2.352725658112587e+102;
et467 = t4.*t12.*t16.*4.39016585121106e+99;
et468 = t5.*t9.*t18.*7.385409687740441e+106;
et469 = t5.*t10.*t17.*-2.406737159744775e+104;
et470 = t5.*t11.*t16.*-7.058176974337762e+99;
et471 = t6.*t9.*t17.*-2.215622906322132e+104;
et472 = t6.*t10.*t16.*3.980872016845588e+101;
et473 = t7.*t9.*t16.*1.769744831185915e+101;
et474 = t4.*t9.*t20.*7.876685970382575e+108;
et475 = t4.*t10.*t19.*-8.086730929592777e+106;
et476 = t4.*t11.*t18.*1.048364122031955e+104;
et477 = t4.*t13.*t16.*1.453481589656482e+98;
et478 = t5.*t9.*t19.*-3.094445352572459e+107;
et479 = t5.*t10.*t18.*1.583854181100554e+105;
et480 = t5.*t11.*t17.*-3.879759733712807e+101;
et481 = t6.*t9.*t18.*1.898957975988716e+105;
et482 = t6.*t10.*t17.*-4.751562543301662e+102;
et483 = t6.*t11.*t16.*9.435277098287593e+98;
et484 = t7.*t9.*t17.*-2.785000817315213e+102;
et485 = t7.*t10.*t16.*2.18341735099005e+99;
et486 = t8.*t9.*t16.*6.380115636009885e+98;
et487 = t5.*t9.*t20.*4.20089918420404e+107;
et488 = t5.*t10.*t19.*-3.234692371837111e+105;
et489 = t5.*t11.*t18.*2.795637658751879e+102;
et490 = t6.*t9.*t19.*-8.079295338036735e+105;
et491 = t6.*t10.*t18.*2.79686382053947e+103;
et492 = t6.*t11.*t17.*-8.386912976255638e+99;
et493 = t7.*t9.*t18.*2.423788601411021e+103;
et494 = t7.*t10.*t17.*-2.9112231346534e+100;
et495 = t8.*t9.*t17.*-1.134242779735091e+100;
et496 = t6.*t9.*t20.*1.260269755261212e+106;
et497 = t6.*t10.*t19.*-6.469384743674221e+103;
et498 = t6.*t11.*t18.*2.795637658751879e+100;
et499 = t7.*t9.*t19.*-1.100040738936975e+104;
et500 = t7.*t10.*t18.*1.940815423102266e+101;
et501 = t8.*t9.*t18.*1.134242779735091e+101;
et502 = t7.*t9.*t20.*2.016431608417939e+104;
et503 = t7.*t10.*t19.*-5.175507794939377e+101;
et504 = t8.*t9.*t19.*-6.049294825253817e+101;
et505 = t9.*t11.*t16.*-8.327804487083089e+104;
et506 = t8.*t9.*t20.*1.344287738945293e+102;
et507 = t9.*t11.*t17.*2.201305295351498e+105;
et508 = t9.*t12.*t16.*2.743853657006913e+102;
et509 = t10.*t11.*t16.*-3.925975719384328e+104;
et510 = t9.*t11.*t18.*1.092045960449953e+106;
et511 = t9.*t13.*t16.*9.084259935353014e+100;
et512 = t10.*t11.*t17.*-5.045252337278782e+104;
et513 = t10.*t12.*t16.*-1.733065408144539e+103;
et514 = t10.*t12.*t17.*-2.227153942375741e+103;
et515 = t2.*t4.*tau.*1.7795489937585e+101;
et516 = t2.*t5.*tau.*1.482726959504415e+100;
et517 = t2.*t6.*tau.*9.802640366977658e+97;
et518 = t2.*t7.*tau.*1.626476838678317e+95;
et519 = t4.*t9.*tau.*-1.160078123616867e+101;
et520 = t4.*t10.*tau.*-4.493508116679646e+101;
et521 = t5.*t9.*tau.*-8.976053632943116e+98;
et522 = t5.*t10.*tau.*-2.958376393959388e+98;
et523 = t6.*t9.*tau.*1.335879643501124e+97;
et524 = t6.*t10.*tau.*3.587004912073848e+97;
et525 = t7.*t10.*tau.*1.626476838678317e+95;
et526 = t2.*t16.*tau.*1.977276659731667e+106;
et527 = t2.*t17.*tau.*-5.491581331497833e+107;
et528 = t2.*t18.*tau.*1.210202514441686e+108;
et529 = t4.*t16.*tau.*9.055989885583628e+103;
et530 = t2.*t19.*tau.*-6.693320323779081e+107;
et531 = t4.*t17.*tau.*3.55314298956999e+103;
et532 = t5.*t16.*tau.*-1.065942896870997e+101;
et533 = t4.*t18.*tau.*1.583264762667999e+105;
et534 = t5.*t17.*tau.*-5.859306652062664e+102;
et535 = t6.*t16.*tau.*1.424938286401199e+100;
et536 = t5.*t18.*tau.*4.222039367114664e+103;
et537 = t6.*t17.*tau.*-1.266611810134399e+101;
et538 = t6.*t18.*tau.*4.222039367114664e+101;
et539 = t9.*t16.*tau.*-1.28897569290763e+106;
et540 = t9.*t17.*tau.*3.32446430849745e+106;
et541 = t10.*t16.*tau.*-4.992786796310718e+106;
et542 = t9.*t18.*tau.*1.649234127779166e+107;
et543 = t10.*t17.*tau.*1.095694960725699e+106;
et544 = t10.*t18.*tau.*4.428401126017097e+107;
et545 = t10.*t19.*tau.*-6.693320323779081e+107;
et546 = t2.*t4.*z.*-1.495407179192811e+104;
et547 = t2.*t5.*z.*-5.444732787290984e+102;
et548 = t2.*t6.*z.*-4.152477703546651e+100;
et549 = t2.*t7.*z.*-8.187815066212686e+97;
et550 = t2.*t11.*z.*1.485296829226032e+104;
et551 = t4.*t9.*z.*2.898740454417078e+105;
et552 = t2.*t12.*z.*6.486203244649786e+102;
et553 = t4.*t10.*z.*8.965273848802465e+103;
et554 = t5.*t9.*z.*2.006767787886949e+103;
et555 = t2.*t13.*z.*-6.994880150221821e+99;
et556 = t4.*t11.*z.*-1.121054445435647e+102;
et557 = t5.*t10.*z.*-2.510764207698172e+101;
et558 = t6.*t9.*z.*-4.46626787231598e+101;
et559 = t2.*t14.*z.*-1.852673427797059e+98;
et560 = t4.*t12.*z.*-6.585248776816591e+98;
et561 = t5.*t11.*z.*2.88818254764723e+99;
et562 = t6.*t10.*z.*-1.649277047330599e+100;
et563 = t7.*t9.*z.*-5.918780107896071e+99;
et564 = t4.*t13.*z.*-2.180222384484723e+97;
et565 = t6.*t11.*z.*-4.717638549143796e+97;
et566 = t7.*t10.*z.*-8.187815066212686e+97;
et567 = t8.*t9.*z.*-1.914034690802966e+97;
et568 = t9.*t11.*z.*-3.71712466691834e+104;
et569 = t9.*t12.*z.*3.748515673519994e+101;
et570 = t10.*t11.*z.*-7.845455447035646e+103;
et571 = t9.*t13.*z.*1.241046171068252e+100;
et572 = t10.*t12.*z.*-3.533688831542073e+102;
et573 = t10.*t13.*z.*-6.994880150221821e+99;
et574 = t10.*t14.*z.*-1.852673427797059e+98;
et575 = tau.*z.*t2.*2.772852976097078e+106;
et576 = t4.*tau.*z.*-1.685533699486763e+103;
et577 = t5.*tau.*z.*4.361802888656245e+100;
et578 = t6.*tau.*z.*-7.124691432005995e+98;
et579 = t9.*tau.*z.*-5.656438893201455e+105;
et580 = t10.*tau.*z.*1.047632706106703e+105;
et581 = mass_l.*t2.*t11.*t16.*-1.529871866233045e+103;
et582 = mass_l.*t2.*t11.*t17.*-6.054302804734539e+103;
et583 = mass_l.*t2.*t12.*t16.*-6.753398899465959e+101;
et584 = mass_l.*t2.*t12.*t17.*-2.672584730850889e+102;
et585 = mass_l.*t9.*t11.*t16.*-8.643418355482819e+103;
et586 = mass_l.*t9.*t11.*t17.*1.331111201881854e+104;
et587 = mass_l.*t9.*t12.*t16.*2.19508292560553e+101;
et588 = mass_l.*t10.*t11.*t16.*-2.686707865152372e+103;
et589 = mass_l.*t9.*t11.*t18.*1.747273536719925e+105;
et590 = mass_l.*t9.*t13.*t16.*7.267407948282412e+99;
et591 = mass_l.*t10.*t11.*t17.*-6.054302804734539e+103;
et592 = mass_l.*t10.*t12.*t16.*-1.186008471701814e+102;
et593 = mass_l.*t10.*t12.*t17.*-2.672584730850889e+102;
et594 = mass_l.*t2.*t16.*tau.*6.524244526133383e+105;
et595 = mass_l.*t2.*t17.*tau.*-8.042140615127423e+106;
et596 = mass_l.*t2.*t18.*tau.*2.036723827963384e+107;
et597 = mass_l.*t2.*t19.*tau.*-1.338664064755816e+107;
et598 = mass_l.*t9.*t16.*tau.*-1.330382342090875e+105;
et599 = mass_l.*t9.*t17.*tau.*2.010276216861942e+105;
et600 = mass_l.*t10.*t16.*tau.*-4.092841983513888e+105;
et601 = mass_l.*t9.*t18.*tau.*2.638774604446665e+106;
et602 = mass_l.*t10.*t17.*tau.*-3.999247398349677e+105;
et603 = mass_l.*t10.*t18.*tau.*8.089439850194217e+106;
et604 = mass_l.*t10.*t19.*tau.*-1.338664064755816e+107;
et605 = mass_l.*t2.*t11.*z.*7.429145749345232e+102;
et606 = mass_l.*t2.*t12.*z.*3.251319106430224e+101;
et607 = mass_l.*t2.*t13.*z.*-2.797952060088728e+98;
et608 = mass_l.*t2.*t14.*z.*-7.410693711188237e+96;
et609 = mass_l.*t9.*t11.*z.*-9.871815975423508e+102;
et610 = mass_l.*t9.*t12.*z.*-1.469059247961501e+99;
et611 = mass_l.*t10.*t11.*z.*-7.82596747183662e+101;
et612 = mass_l.*t9.*t13.*z.*-4.863712769388004e+97;
et613 = mass_l.*t10.*t12.*z.*-3.73636287730106e+100;
et614 = mass_l.*t10.*t13.*z.*-2.797952060088728e+98;
et615 = mass_l.*t10.*t14.*z.*-7.410693711188237e+96;
et616 = mass_l.*tau.*z.*t2.*9.905045908549313e+104;
et617 = mass_l.*t9.*tau.*z.*-1.489190141536004e+104;
et618 = mass_l.*t10.*tau.*z.*3.414725160229112e+104;
et619 = t2.*t4.*t11.*t16.*-3.353074703355479e+100;
et620 = t2.*t4.*t11.*t17.*-2.421721121893816e+102;
et621 = t2.*t4.*t12.*t16.*-1.480166510102917e+99;
et622 = t2.*t5.*t11.*t16.*7.265163365681447e+99;
et623 = t2.*t4.*t12.*t17.*-1.069033892340356e+101;
et624 = t2.*t5.*t11.*t17.*-3.228961495858421e+100;
et625 = t2.*t5.*t12.*t16.*3.207101677021067e+98;
et626 = t2.*t5.*t12.*t17.*-1.425378523120474e+99;
et627 = t4.*t9.*t11.*t16.*-2.327683711943398e+102;
et628 = t4.*t9.*t11.*t17.*-5.15919641279213e+102;
et629 = t4.*t9.*t12.*t16.*4.39016585121106e+99;
et630 = t4.*t10.*t11.*t16.*-2.648979468174201e+101;
et631 = t5.*t9.*t11.*t16.*1.547758923837639e+100;
et632 = t4.*t9.*t11.*t18.*1.048364122031955e+104;
et633 = t4.*t9.*t13.*t16.*1.453481589656482e+98;
et634 = t4.*t10.*t11.*t17.*-2.421721121893816e+102;
et635 = t4.*t10.*t12.*t16.*-1.169353814520728e+100;
et636 = t5.*t9.*t11.*t17.*-4.88134934316677e+101;
et637 = t5.*t10.*t11.*t16.*7.265163365681447e+99;
et638 = t6.*t9.*t11.*t16.*9.435277098287593e+98;
et639 = t4.*t10.*t12.*t17.*-1.069033892340356e+101;
et640 = t5.*t9.*t11.*t18.*2.795637658751879e+102;
et641 = t5.*t10.*t11.*t17.*-3.228961495858421e+100;
et642 = t5.*t10.*t12.*t16.*3.207101677021067e+98;
et643 = t6.*t9.*t11.*t17.*-8.386912976255638e+99;
et644 = t5.*t10.*t12.*t17.*-1.425378523120474e+99;
et645 = t6.*t9.*t11.*t18.*2.795637658751879e+100;
et646 = t2.*t4.*t16.*tau.*4.923812182034017e+104;
et647 = t2.*t4.*t17.*tau.*-4.438890542829e+105;
et648 = t2.*t5.*t16.*tau.*1.3316671628487e+103;
et649 = t2.*t4.*t18.*tau.*1.322434101634717e+106;
et650 = t2.*t5.*t17.*tau.*-1.120825713031087e+104;
et651 = t2.*t6.*t16.*tau.*1.190190691471245e+101;
et652 = t2.*t4.*t19.*tau.*-1.070931251804653e+106;
et653 = t2.*t5.*t18.*tau.*4.061956563594904e+104;
et654 = t2.*t6.*t17.*tau.*-1.218586969078471e+102;
et655 = t2.*t7.*t16.*tau.*2.891514379872563e+98;
et656 = t2.*t5.*t19.*tau.*-4.283725007218612e+104;
et657 = t2.*t6.*t18.*tau.*5.668353441301884e+102;
et658 = t2.*t7.*t17.*tau.*-3.855352506496751e+99;
et659 = t2.*t6.*t19.*tau.*-8.567450014437224e+102;
et660 = t2.*t7.*t18.*tau.*2.570235004331167e+100;
et661 = t2.*t7.*t19.*tau.*-6.853960011549779e+100;
et662 = t4.*t9.*t16.*tau.*-3.565388981769623e+103;
et663 = t4.*t9.*t17.*tau.*-7.791542759232223e+103;
et664 = t4.*t10.*t16.*tau.*-6.38602263777042e+103;
et665 = t5.*t9.*t16.*tau.*2.337462827769667e+101;
et666 = t4.*t9.*t18.*tau.*1.583264762667999e+105;
et667 = t4.*t10.*t17.*tau.*-6.453362869456401e+104;
et668 = t5.*t9.*t17.*tau.*-7.371931418569626e+102;
et669 = t5.*t10.*t16.*tau.*1.93600886083692e+102;
et670 = t6.*t9.*t16.*tau.*1.424938286401199e+100;
et671 = t4.*t10.*t18.*tau.*5.857661958683392e+105;
et672 = t5.*t9.*t18.*tau.*4.222039367114664e+103;
et673 = t5.*t10.*t17.*tau.*-3.203513166067544e+103;
et674 = t6.*t9.*t17.*tau.*-1.266611810134399e+101;
et675 = t6.*t10.*t16.*tau.*5.271895762815053e+100;
et676 = t4.*t10.*t19.*tau.*-1.070931251804653e+106;
et677 = t5.*t10.*t18.*tau.*2.097508814884564e+104;
et678 = t6.*t9.*t18.*tau.*4.222039367114664e+101;
et679 = t6.*t10.*t17.*tau.*-6.292526444653693e+101;
et680 = t7.*t10.*t16.*tau.*2.891514379872563e+98;
et681 = t5.*t10.*t19.*tau.*-4.283725007218612e+104;
et682 = t6.*t10.*t18.*tau.*3.703905692591544e+102;
et683 = t7.*t10.*t17.*tau.*-3.855352506496751e+99;
et684 = t6.*t10.*t19.*tau.*-8.567450014437224e+102;
et685 = t7.*t10.*t18.*tau.*2.570235004331167e+100;
et686 = t7.*t10.*t19.*tau.*-6.853960011549779e+100;
et687 = t2.*t4.*t11.*z.*4.589615598699135e+100;
et688 = t2.*t4.*t12.*z.*2.026019669839788e+99;
et689 = t2.*t5.*t11.*z.*-5.448872524261085e+98;
et690 = t2.*t5.*t12.*z.*-2.4053262577658e+97;
et691 = t4.*t9.*t11.*z.*2.593025506644846e+101;
et692 = t4.*t9.*t12.*z.*-6.585248776816591e+98;
et693 = t4.*t10.*t11.*z.*8.060123595457115e+100;
et694 = t5.*t9.*t11.*z.*1.198000081693669e+99;
et695 = t4.*t9.*t13.*z.*-2.180222384484723e+97;
et696 = t4.*t10.*t12.*z.*3.558025415105443e+99;
et697 = t5.*t10.*t11.*z.*-5.448872524261085e+98;
et698 = t6.*t9.*t11.*z.*-4.717638549143796e+97;
et699 = t5.*t10.*t12.*z.*-2.4053262577658e+97;
et700 = t2.*t4.*tau.*z.*-1.957273357840015e+103;
et701 = t2.*t5.*tau.*z.*-7.237926553614681e+101;
et702 = t2.*t6.*tau.*z.*-5.499154335501137e+99;
et703 = t2.*t7.*tau.*z.*-1.084317892452211e+97;
et704 = t4.*t9.*tau.*z.*3.991147026272625e+102;
et705 = t4.*t10.*tau.*z.*1.227852595054166e+103;
et706 = t5.*t9.*tau.*z.*1.809248595175747e+100;
et707 = t5.*t10.*tau.*z.*-3.599322658514709e+100;
et708 = t6.*t9.*tau.*z.*-7.124691432005995e+98;
et709 = t6.*t10.*tau.*z.*-2.184148759552439e+99;
et710 = t7.*t10.*tau.*z.*-1.084317892452211e+97;
et711 = -1.434957421705908e+107;
et712 = et257+et258+et259+et260+et261+et262+et263+et264+et265+et266+et267+et268+et269+et270+et271+et272+et273+et274+et275+et276+et277+et278+et279+et280+et281+et282+et283+et284+et285+et286+et287+et288+et289+et290+et291+et292+et293+et294+et295+et296+et297+et298+et299+et300+et301+et302+et303+et304+et305+et306+et307+et308+et309+et310+et311+et312+et313+et314+et315+et316+et317+et318+et319+et320+et321+et322+et323+et324+et325+et326+et327+et328+et329+et330+et331+et332+et333+et334+et335+et336+et337+et338+et339+et340+et341+et342+et343+et344+et345+et346+et347+et348+et349+et350+et351+et352+et353+et354+et355+et356+et357+et358+et359+et360+et361+et362+et363+et364+et365+et366+et367+et368+et369+et370+et371+et372+et373+et374+et375+et376+et377+et378+et379+et380+et381+et382+et383+et384+et385+et386+et387+et388+et389+et390+et391+et392+et393+et394+et395+et396+et397+et398+et399+et400+et401+et402+et403+et404+et405+et406+et407+et408+et409+et410+et411+et412+et413+et414+et415+et416+et417+et418+et419+et420+et421+et422+et423+et424+et425+et426+et427+et428+et429+et430+et431+et432+et433+et434+et435+et436+et437+et438+et439+et440+et441+et442+et443+et444+et445+et446+et447+et448+et449+et450+et451+et452+et453+et454+et455+et456;
et713 = et457+et458+et459+et460+et461+et462+et463+et464+et465+et466+et467+et468+et469+et470+et471+et472+et473+et474+et475+et476+et477+et478+et479+et480+et481+et482+et483+et484+et485+et486+et487+et488+et489+et490+et491+et492+et493+et494+et495+et496+et497+et498+et499+et500+et501+et502+et503+et504+et505+et506+et507+et508+et509+et510+et511+et512+et513+et514+et515+et516+et517+et518+et519+et520+et521+et522+et523+et524+et525+et526+et527+et528+et529+et530+et531+et532+et533+et534+et535+et536+et537+et538+et539+et540+et541+et542+et543+et544+et545+et546+et547+et548+et549+et550+et551+et552+et553+et554+et555+et556+et557+et558+et559+et560+et561+et562+et563+et564+et565+et566+et567+et568+et569+et570+et571+et572+et573+et574+et575+et576+et577+et578+et579+et580+et581+et582+et583+et584+et585+et586+et587+et588+et589+et590+et591+et592+et593+et594+et595+et596+et597+et598+et599+et600+et601+et602+et603+et604+et605+et606+et607+et608+et609+et610+et611+et612+et613+et614+et615+et616+et617+et618+et619+et620+et621+et622+et623+et624+et625+et626+et627+et628+et629+et630+et631+et632+et633+et634+et635+et636+et637+et638+et639+et640+et641+et642+et643+et644+et645+et646+et647+et648+et649+et650+et651+et652+et653+et654+et655+et656;
et714 = et657+et658+et659+et660+et661+et662+et663+et664+et665+et666+et667+et668+et669+et670+et671+et672+et673+et674+et675+et676+et677+et678+et679+et680+et681+et682+et683+et684+et685+et686+et687+et688+et689+et690+et691+et692+et693+et694+et695+et696+et697+et698+et699+et700+et701+et702+et703+et704+et705+et706+et707+et708+et709+et710+et711;
ik_ddelta2 = dz.*t211.*(et712+et713+et714).*5.520653160719109e+15;
if nargout > 4
    ik_lt = sqrt(t33.*(t24.*1.7102875e+1+mass_l.*t24.*(1.59e+2./4.0e+2)-t24.*t209.*2.5e+1-mass_l.*t24.*t209).^2+t33.*(t25.*1.7102875e+1+tau.*1.019716212977928e-1+mass_l.*t25.*(1.59e+2./4.0e+2)-t25.*t209.*2.5e+1-mass_l.*t25.*t209+7.7e+1./1.0e+2).^2);
end
end
